simulink model "FanControl"  (R2024a)
settings: Solver=FixedStepDiscrete  StartTime=0.01  StopTime=0.1  RelTol=1e-3
settings Model: Creator=Hakima Ayed  LastModifiedBy=Hakima Ayed
settings OptimizationCC: DefaultParameterBehavior=Inlined  EnhancedBackFolding=on  PassReuseOutputArgsAs=Individual arguments  ZeroExternalMemoryAtStartup=off  ZeroInternalMemoryAtStartup=off  OptimizeBlockOrder=speed  DifferentSizesBufferReuse=on  OptimizationCustomize=off  EfficientTunableParamExpr=on
settings DebuggingCC: ParameterTunabilityLossMsg=error
settings SFSimCC: MATLABDynamicMemAlloc=off
settings RTWCC: Description=Embedded Coder  SystemTargetFile=ert.tlc  TemplateMakefile=ert_default_tmf
settings CodeAppCC: ForceParamTrailComments=on  IgnoreCustomStorageClasses=off  OperatorAnnotations=on  SimulinkDataObjDesc=on  SFDataObjDesc=on  InsertBlockDesc=on
settings ERTTargetCC: TargetLangStandard=C99 (ISO)  GenerateSampleERTMain=on  InlinedParameterPlacement=NonHierarchical  ERTCustomFileTemplate=example_file_process.tlc

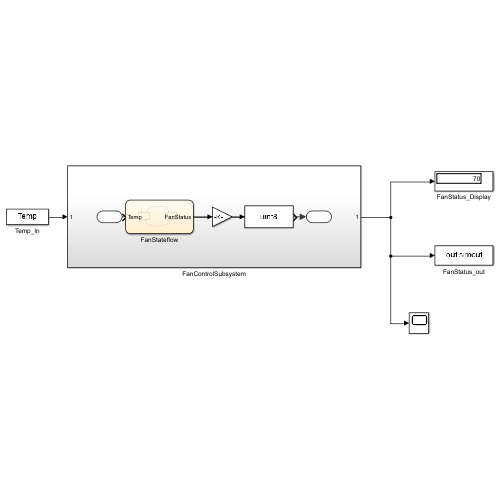
[thumbnail: Simulink's stored preview of the top-level diagram]
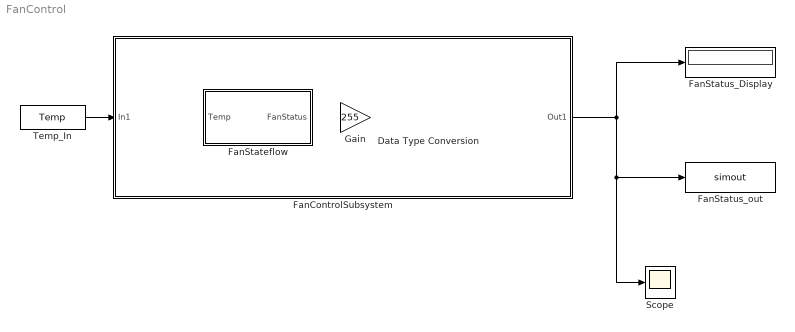
== system FanControl ==
  Data Type Conversion : DataTypeConversion  OutDataTypeStr=uint8  SaturateOnIntegerOverflow=off  RndMeth=Floor
  FanControlSubsystem : Subsystem
  FanStateflow : Stateflow chart  TreatAsAtomicUnit=on
  FanStatus_Display : Display
  FanStatus_out : ToWorkspace  VariableName=simout  SaveFormat=Timeseries  SampleTime=-1
  Gain : Gain  Gain=255
  Scope : Scope
  Temp_In : FromWorkspace  VariableName=Temp
  wires:
  Temp_In/1 -> FanControlSubsystem/1(In1)
  FanControlSubsystem/1(Out1) -> Scope/1, FanStatus_out/1, FanStatus_Display/1
  FanStateflow/1(FanStatus) -> Gain/1
  Gain/1 -> Data Type Conversion/1

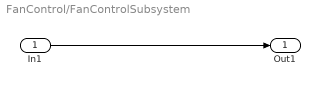
== system FanControl/FanControlSubsystem ==
  In1 : Inport
  Out1 : Outport
  wires:
  In1/1 -> Out1/1

== stateflow chart FanControl/FanStateflow ==
  state Fan_OFF
    during :FanStatus=0;
  state Fan_ON
    during :FanStatus=1;
  Fan_OFF -> Fan_ON : [ Temp > 90 ]
  (default) -> Fan_OFF
  Fan_ON -> Fan_OFF : [ Temp < 80 ]
  data: Temp input double; FanStatus output uint8
